simulink model "ThyroidCheckupV1"  (R2022a)
settings: Solver=VariableStepAuto  StartTime=0.0  StopTime=10.0  RelTol=1e-3
libraries: simulink x5
settings Model: Creator=NEMALI MAHESH  LastModifiedBy=NEMALI MAHESH

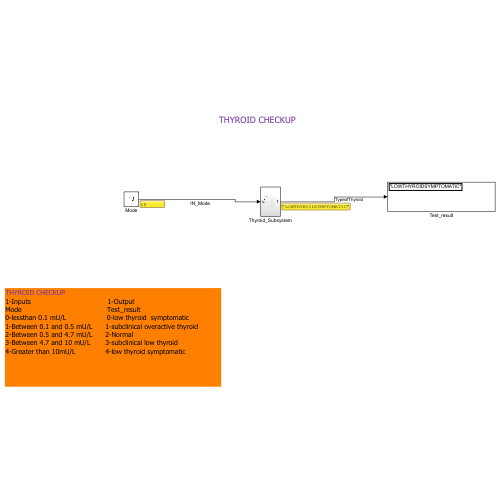
[thumbnail: Simulink's stored preview of the top-level diagram]
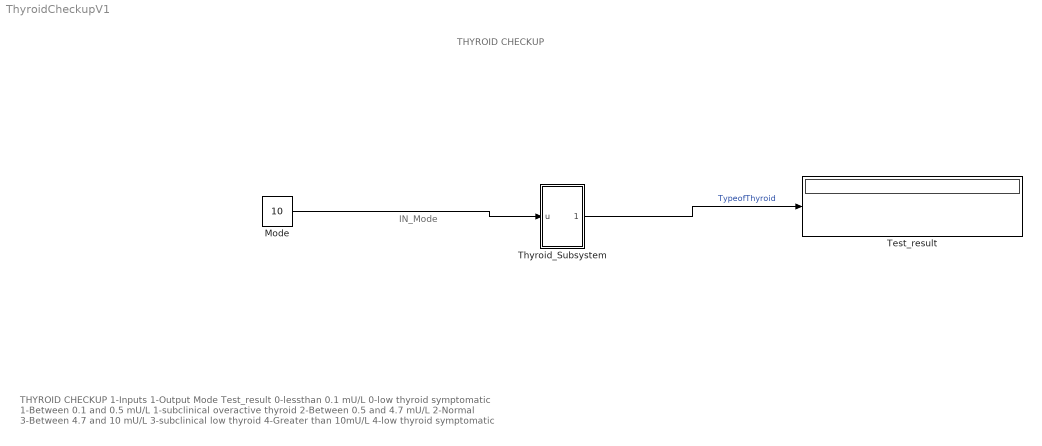
== system ThyroidCheckupV1 ==
  note: THYROID CHECKUP
      | 1-Inputs 1-Output
      | Mode Test_result
      | 0-lessthan 0.1 mU/L 0-low thyroid symptomatic
      | 1-Between 0.1 and 0.5 mU/L 1-subclinical overactive thyroid
      | 2-Between 0.5 and 4.7 mU/L 2-Normal
      | 3-Between 4.7 and 10 mU/L 3-subclinical low thyroid
      | 4-Greater than 10mU/L 4-low thyroid symptomatic
  note: THYROID CHECKUP
  note: IN_Mode
  Mode : Constant  Value=10
  Test_result : Display
  Thyroid_Subsystem : Subsystem
  wires:
  Mode/1 -> Thyroid_Subsystem/1(u)
  Thyroid_Subsystem/1(Out1) -> Test_result/1  "TypeofThyroid"

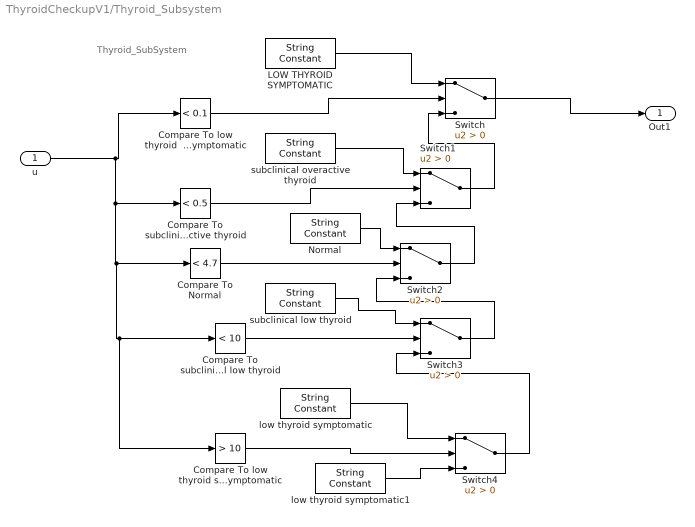
== system ThyroidCheckupV1/Thyroid_Subsystem ==
  note: Thyroid_SubSystem
  u : Inport
  Compare To Normal : simulink/Logic and Bit Operations/Compare To Constant  relop=<  const=4.7  OutDataTypeStr=boolean
  Compare To low thyroid  symptomatic : simulink/Logic and Bit Operations/Compare To Constant  relop=<  const=0.1  OutDataTypeStr=boolean
  Compare To low thyroid symptomatic : simulink/Logic and Bit Operations/Compare To Constant  relop=>  const=10  OutDataTypeStr=boolean
  "Compare To subclinical low thyroid " : simulink/Logic and Bit Operations/Compare To Constant  relop=<  const=10  OutDataTypeStr=boolean
  Compare To subclinical overactive thyroid : simulink/Logic and Bit Operations/Compare To Constant  relop=<  const=0.5  OutDataTypeStr=boolean
  LOW THYROID SYMPTOMATIC : StringConstant  String="\"LOW THYROID SYMPTOMATIC\""
  Normal : StringConstant  String="\"NORMAL\""
  Switch{,1..4} (5 alike) : Switch  Criteria=u2 > Threshold  SaturateOnIntegerOverflow=off  InputSameDT=off
  low thyroid symptomatic : StringConstant  String="\"LOWTHYROIDSYMPTOMATIC\""
  low thyroid symptomatic1 : StringConstant  String="\"LOWTHYROIDSYMPTOMATIC\""
  subclinical low thyroid : StringConstant  String="\"SUBCLINICAL LOW THYROID\""
  subclinical overactive thyroid : StringConstant  String="\"SUBCLINICAL OVERACTIVE \""
  Out1 : Outport
  wires:
  Normal/1 -> Switch2/1
  subclinical low thyroid/1 -> Switch3/1
  Compare To Normal/1 -> Switch2/2
  LOW THYROID SYMPTOMATIC/1 -> Switch/1
  Switch/1 -> Out1/1
  low thyroid symptomatic/1 -> Switch4/1
  Switch3/1 -> Switch2/3
  u/1 -> Compare To low thyroid symptomatic/1, "Compare To subclinical low thyroid "/1, Compare To Normal/1, Compare To subclinical overactive thyroid/1, Compare To low thyroid  symptomatic/1
  Switch1/1 -> Switch/3
  Compare To low thyroid symptomatic/1 -> Switch4/2
  Compare To low thyroid  symptomatic/1 -> Switch/2
  Compare To subclinical overactive thyroid/1 -> Switch1/2
  Switch2/1 -> Switch1/3
  Switch4/1 -> Switch3/3
  "Compare To subclinical low thyroid "/1 -> Switch3/2
  subclinical overactive thyroid/1 -> Switch1/1
  low thyroid symptomatic1/1 -> Switch4/3
